simulink model "robosim"  (Simulink 8.9)
settings: Solver=ode45  StartTime=0.0  StopTime=5  MaxStep=0.1  RelTol=1e-4  EnableMultiTasking=on
values from neighbouring files (symbols this model uses):
  ki = (c * b)^2 / k    (= 625000)    [ex.m]
  kp1 = b*(2*c - c^2 - 1)/(c*(c-2))    (= 18)    [ex.m]
  kp2 = - 2 * c * b / k    (= 50000)    [ex.m]
undefined symbols (not defined in the file): q0
settings Model: SuppressorTable=22 serialization::archive 11 0 6 0 0 0 11 0  Creator=fernando  LastModifiedBy=rbp  ExtModeAutoUpdateStatusClock=off
settings OptimizationCC: ExpressionDepthLimit=2147483647  InitFltsAndDblsToZero=on
settings DebuggingCC: SaveWithParameterizedLinksMsg=none  SignalResolutionControl=TryResolveAllWithWarning  SolverPrmCheckMsg=warning  MultiTaskDSMMsg=warning  MultiTaskCondExecSysMsg=none
settings SFSimCC: SimParseCustomCode=off
settings GRTTargetCC: TargetFcnLib=ansi_tfl_tmw.mat

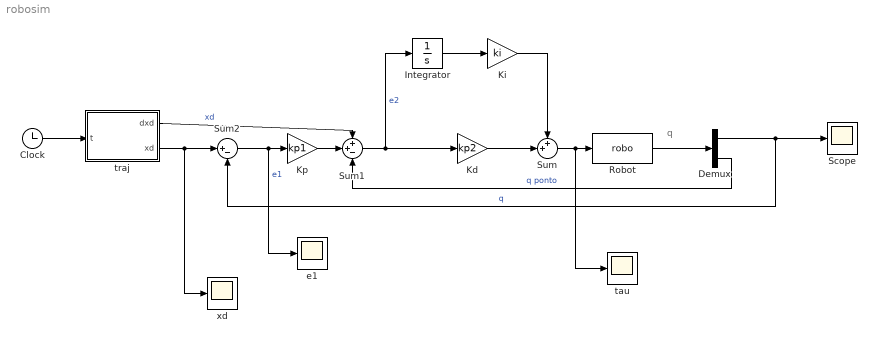
== system robosim ==
  note: q
  Clock : Clock
  Demux : Demux  Outputs=2
  Integrator : Integrator
  Kd : Gain  Gain=kp2
  Ki : Gain  Gain=ki
  Kp : Gain  Gain=kp1
  Robot : S-Function  FunctionName=robo  Parameters=q0  SFunctionDeploymentMode=off  EnableBusSupport=off  mask(Robot){xi=q0}
      mask prompts: xi "Condicao Inicial"
  Scope : Scope
  Sum : Sum  Inputs=++|
  Sum1 : Sum  Inputs=++-
  Sum2 : Sum  Inputs=|+-
  e1 : Scope
  tau : Scope
  traj : MATLAB Function  TreatAsAtomicUnit=on
  xd : Scope
  wires:
  Demux/1 -> Sum2/2, Scope/1  "q"
  Robot/1 -> Demux/1
  Sum/1 -> tau/1, Robot/1
  Ki/1 -> Sum/1
  Kd/1 -> Sum/2
  Sum1/1 -> Integrator/1, Kd/1  "e2"
  Sum2/1 -> e1/1, Kp/1  "e1"
  Kp/1 -> Sum1/2
  Demux/2 -> Sum1/3  "q ponto"
  traj/2(xd) -> xd/1, Sum2/1
  traj/1(dxd) -> Sum1/1  "xd"
  Clock/1 -> traj/1(t)
  Integrator/1 -> Ki/1

== matlab function traj ==
  data: t input double; dxd output double; xd output double
function [dxd, xd] = traj(t)

    xd = xdFunc(t);
    dxd = dxdFunc(t);

end
